simulink model "Lombardini_dual_fuel"  (R2024b)
settings: Solver=FixedStepAuto  StartTime=0.0  StopTime=2000  RelTol=1e-3  EnableMultiTasking=on
PreLoadFcn:
  | try, eval([bdroot '_setup']); catch, eval('model_setup', ''); end
InitFcn:
  | try, eval([bdroot '_setup']); catch, eval('model_setup', ''); end
model workspace (MAT data in the model file):
  PID_rpm = [1000 2000 3000 4000]
undefined symbols (not defined in the file): ECU555, motohawk_build_version, motohawk_get_target_image, motohawk_target_type, motohawk_trunc_name, motohawk_vardec_path
libraries: MotoHawk_lib x118, motohawk_annotations_lib x23, dspstat3 x13, motohawk_examples_lib x1, MotoHawk_Protocols_lib x1
(part 5 of 5)

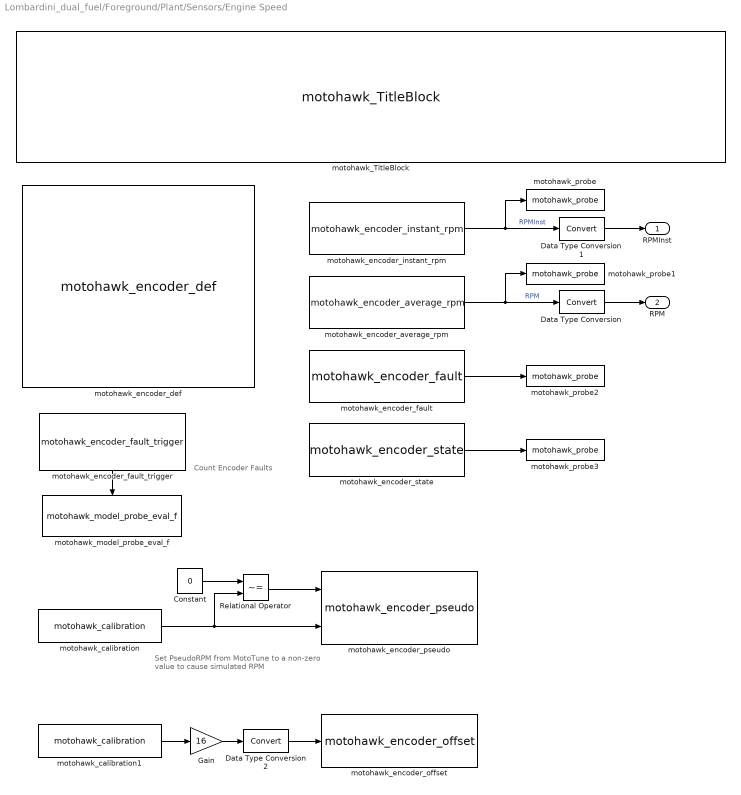
== system Lombardini_dual_fuel/Foreground/Plant/Sensors/Engine Speed ==
  note: Set PseudoRPM from MotoTune
      | to a non-zero value to cause
      | simulated RPM
  note: Count
      | Encoder
      | Faults
  Constant : Constant  Value=0  OutDataTypeStr=Inherit: Inherit via back propagation
  Data Type Conversion : DataTypeConversion
  Data Type Conversion1 : DataTypeConversion
  Data Type Conversion2 : DataTypeConversion
  Gain : Gain  Gain=16  OutDataTypeStr=Inherit: Same as input  ParamDataTypeStr=Inherit: Same as input
  Relational Operator : RelationalOperator  Operator=~=  ZeroCross=off
  motohawk_TitleBlock : motohawk_annotations_lib/motohawk_TitleBlock  BlockType_='Mototron_Title_Block'  ttl=[get_param(bdroot, 'Description') '\rm\newlineEngine Encoder Interface\newlineOutput RPM for use in the controller\newline']  copyright="'THE INFORMATION CONTAINED IN THIS\\newlineDRAWING IS THE SOLE PROPERTY OF\\newlineWOODWARD.  ANY REPRODUCTION IN\\newline PART OR AS A WHOLE WITHOUT THE\\newlineWRITTEN PERMISSION OF WOODWARD\\newline IS PROHIBITED.\\fontsize{16}\\rm\\copyright\\rm\\fontsize{10} 2017'"  address='\fontsize{22}\it\fontname{Arial Black}Woodward \fontname{Arial}\fontsize{10}\newline1081 Woodward Way, Fort Collins, CO, 80524\newlinemcs.woodward.com'  image_file='mh.jpg'  pretty_print=on  edit_text=|  edit_as=6
      | [get_param(bdroot, 'Description') '\rm
      | 
      | 
      | Engine Encoder Interface
      | 
      | 
      | Output RPM for use in the controller
      | 
      | 
      | ']
      settings: SourceProductName=MotoHawk Annotations
  motohawk_calibration : MotoHawk_lib/Calibration & Probing Blocks/motohawk_calibration  name_source=Use Parameter  nam='PseudoRPM'  val=0  storage=Display  ovr_cals=on  data_type=Inherit via back propagation  mem_region_use=off  mem_region_name='SERIAL_EE'  read_level=1  write_level=1  view_as=Number  enum_struct={'Disabled', 'Enabled'}  vector_style=Wide Row  row_header_enum={}  col_header_enum={}  mototune_group=motohawk_vardec_path(gcb)  help=''  units=''  min_val=-inf  max_val=inf  precision=''  gain=1  offset=0  exp=1  show_more=on  use_help_units=off  use_header_enum=off  use_min_max=off  use_precision=off  use_mototune_group=off  data_stores=motohawk_sfun_calibration_data_stores
      settings: SourceProductName=MotoHawk
  motohawk_calibration1 : MotoHawk_lib/Calibration & Probing Blocks/motohawk_calibration  name_source=Use Parameter  nam='EncoderTDCOffset'  val=0  storage=Calibration  ovr_cals=on  data_type=Inherit via back propagation  mem_region_use=off  mem_region_name='SERIAL_EE'  read_level=1  write_level=1  view_as=Number  enum_struct={'Disabled', 'Enabled'}  vector_style=Wide Row  row_header_enum={}  col_header_enum={}  mototune_group='System | Encoder | Encoder Config'  help="'TDC offset of crank sensor, in degrees before TDC1.  Used to align sensor with crank angle.'"  units='degCA'  min_val=0  max_val=720  precision=''  gain=1  offset=0  exp=1  show_more=on  use_help_units=on  use_header_enum=off  use_min_max=on  use_precision=off  use_mototune_group=on  data_stores=motohawk_sfun_calibration_data_stores
      settings: SourceProductName=MotoHawk
  motohawk_encoder_average_rpm : MotoHawk_lib/Encoder Blocks/motohawk_encoder_average_rpm  resolution=1
      settings: SourceProductName=MotoHawk
  motohawk_encoder_def : MotoHawk_lib/Encoder Blocks/motohawk_encoder_def  encoder_type=60 Minus 6 - 4-Stroke - No CAM  interface=VR Crank  sync=Falling Edge  crnkpullup=Weak Pullup  camsync=Rising Edge  campullup=Weak Pullup  angle_offset=0  sec_tdcoffset=-34.3  cam_delay=0  teeth_after_cam=-1  ignore_teeth=0  ignore_delay=0  angles=[0 360 180 540]  cnk_align_with_cam=off  adaptive_vr_cnk=off  adaptive_vr_cam=on  cal_cylinders=on  max_cylinders=8  num_cylinders=4  read_level=1  write_level=1  ovr_cals=on  group='System | Encoder'
      settings: SourceProductName=MotoHawk
  motohawk_encoder_fault : MotoHawk_lib/Encoder Blocks/motohawk_encoder_fault
      settings: SourceProductName=MotoHawk
  motohawk_encoder_fault_trigger : MotoHawk_lib/Encoder Blocks/motohawk_encoder_fault_trigger  Tag=Trigger  trig_name=[]  use_task_name=off  task_priority=ApplicationInterruptTask  task_name='ApplicationInterruptTask'  inherited=off
      settings: SourceProductName=MotoHawk
  motohawk_encoder_instant_rpm : MotoHawk_lib/Encoder Blocks/motohawk_encoder_instant_rpm  resolution=1
      settings: SourceProductName=MotoHawk
  motohawk_encoder_offset : MotoHawk_lib/Encoder Blocks/motohawk_encoder_offset
      settings: SourceProductName=MotoHawk
  motohawk_encoder_pseudo : MotoHawk_lib/Encoder Blocks/motohawk_encoder_pseudo
      settings: SourceProductName=MotoHawk
  motohawk_encoder_state : MotoHawk_lib/Encoder Blocks/motohawk_encoder_state
      settings: SourceProductName=MotoHawk
  motohawk_model_probe_eval_f : MotoHawk_lib/Extra Development Blocks/motohawk_model_probe_eval_f  nam='EncoderFaultCount'  group=motohawk_vardec_path(gcb)
      settings: SourceProductName=MotoHawk
  motohawk_probe : MotoHawk_lib/Calibration & Probing Blocks/motohawk_probe  nam='RPMInst'  show_more=on  name_source=Use Input Wire Name  read_level=1  view_as=Number  enum_struct={'Disabled', 'Enabled'}  vector_style=Wide Row  use_help_units=off  help=''  units=''  use_header_enum=off  row_header_enum={}  col_header_enum={}  use_min_max=off  min_val=-inf  max_val=inf  use_precision=off  precision=''  gain=1  offset=0  exp=1  use_mototune_group=off  mototune_group=motohawk_vardec_path(gcb)
      settings: SourceProductName=MotoHawk
  motohawk_probe1 : MotoHawk_lib/Calibration & Probing Blocks/motohawk_probe  nam='RPM'  show_more=on  name_source=Use Input Wire Name  read_level=1  view_as=Number  enum_struct={'Disabled', 'Enabled'}  vector_style=Wide Row  use_help_units=off  help=''  units=''  use_header_enum=off  row_header_enum={}  col_header_enum={}  use_min_max=off  min_val=-inf  max_val=inf  use_precision=off  precision=''  gain=1  offset=0  exp=1  use_mototune_group=off  mototune_group=motohawk_vardec_path(gcb)
      settings: SourceProductName=MotoHawk
  motohawk_probe2 : MotoHawk_lib/Calibration & Probing Blocks/motohawk_probe  nam='EncoderFault'  show_more=on  name_source=Use Parameter  read_level=1  view_as=Enumeration  enum_struct={'OK', 'Crank Sync Fault', 'Reverse Rotation', 'No Crank Edges', 'No CAM Edges', 'CAM Sync Fault','Encoder Sync Error on Slave','Reverse Rotation on Slave','Slave Encoder Loss'}  vector_style=Wide Row  use_help_units=on  help='Encoder synchronization fault status'  units=''  use_header_enum=off  row_header_enum={}  col_header_enum={}  use_min_max=off  min_val=-inf  max_val=inf  use_precision=off  precision=''  gain=1  offset=0  exp=1  use_mototune_group=off  mototune_group=motohawk_vardec_path(gcb)
      settings: SourceProductName=MotoHawk
  motohawk_probe3 : MotoHawk_lib/Calibration & Probing Blocks/motohawk_probe  nam='EncoderState'  show_more=on  name_source=Use Parameter  read_level=1  view_as=Enumeration  enum_struct={'', 'Zero Speed', 'Position Unknown', 'Crank Sync - CAM Unknown', 'Crank Sync - CAM Sync', 'Crank Sync - Master Only', 'Crank Sync - Slave Only', 'Crank Sync - Master + Slave'}  vector_style=Wide Row  use_help_units=on  help='Encoder synchronization status'  units=''  use_header_enum=off  row_header_enum={}  col_header_enum={}  use_min_max=off  min_val=-inf  max_val=inf  use_precision=off  precision=''  gain=1  offset=0  exp=1  use_mototune_group=off  mototune_group=motohawk_vardec_path(gcb)
      settings: SourceProductName=MotoHawk
  RPMInst : Outport  VectorParamsAs1DForOutWhenUnconnected=off
  RPM : Outport  Port=2  VectorParamsAs1DForOutWhenUnconnected=off
  wires:
  motohawk_encoder_instant_rpm/1 -> motohawk_probe/1, Data Type Conversion1/1  "RPMInst"
  motohawk_encoder_average_rpm/1 -> motohawk_probe1/1, Data Type Conversion/1  "RPM"
  motohawk_calibration/1 -> motohawk_encoder_pseudo/2, Relational Operator/2
  Relational Operator/1 -> motohawk_encoder_pseudo/1
  Constant/1 -> Relational Operator/1
  Data Type Conversion/1 -> RPM/1
  Data Type Conversion1/1 -> RPMInst/1
  motohawk_encoder_fault/1 -> motohawk_probe2/1
  motohawk_calibration1/1 -> Gain/1
  Gain/1 -> Data Type Conversion2/1
  Data Type Conversion2/1 -> motohawk_encoder_offset/1
  motohawk_encoder_state/1 -> motohawk_probe3/1
  motohawk_encoder_fault_trigger/1 -> motohawk_model_probe_eval_f/Trigger

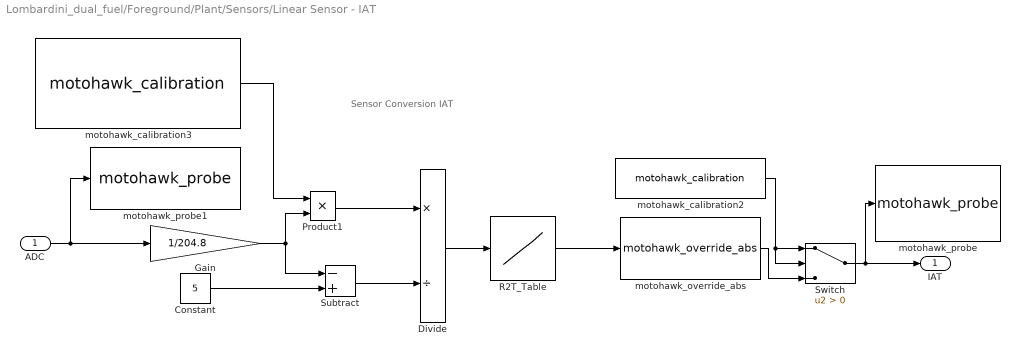
== system Lombardini_dual_fuel/Foreground/Plant/Sensors/Linear Sensor - IAT ==
  note: Sensor Conversion
      | IAT
  ADC : Inport
  Constant : Constant  Value=5
  Divide : Product  Inputs=*/
  Gain : Gain  Gain=1/204.8  OutDataTypeStr=double
  Product1 : Product  InputSameDT=on  OutDataTypeStr=Inherit: Same as first input
  R2T_Table : Lookup_n-D  NumberOfTableDimensions=1  BreakpointsForDimension1=[-5:5]  Table=tanh([-5:5])  InternalRulePriority=Speed  RndMeth=Simplest
  Subtract : Sum  Inputs=-+
  Switch : Switch  Criteria=u2 > Threshold  SaturateOnIntegerOverflow=off  InputSameDT=off
  motohawk_calibration2 : MotoHawk_lib/Calibration & Probing Blocks/motohawk_calibration  name_source=Use Parameter  nam='IAT_Override'  val=25  storage=Calibration  ovr_cals=on  data_type=Inherit from 'Default Value'  mem_region_use=off  mem_region_name='SERIAL_EE'  read_level=1  write_level=1  view_as=Number  enum_struct={'Disabled', 'Enabled'}  vector_style=Wide Row  row_header_enum={}  col_header_enum={}  mototune_group=motohawk_vardec_path(gcb)  help=''  units=''  min_val=-inf  max_val=inf  precision=''  gain=1  offset=0  exp=1  show_more=off  use_help_units=off  use_header_enum=off  use_min_max=off  use_precision=off  use_mototune_group=off  data_stores=motohawk_sfun_calibration_data_stores
      settings: SourceProductName=MotoHawk
  motohawk_calibration3 : MotoHawk_lib/Calibration & Probing Blocks/motohawk_calibration  name_source=Use Parameter  nam='IAT_Calibration_Pullup'  val=1000  storage=Calibration  ovr_cals=on  data_type=Inherit from 'Default Value'  mem_region_use=off  mem_region_name='SERIAL_EE'  read_level=1  write_level=1  view_as=Number  enum_struct={'Disabled', 'Enabled'}  vector_style=Wide Row  row_header_enum={}  col_header_enum={}  mototune_group=motohawk_vardec_path(gcb)  help=''  units=''  min_val=-inf  max_val=inf  precision=''  gain=1  offset=0  exp=1  show_more=off  use_help_units=off  use_header_enum=off  use_min_max=off  use_precision=off  use_mototune_group=off  data_stores=motohawk_sfun_calibration_data_stores
      settings: SourceProductName=MotoHawk
  motohawk_override_abs : MotoHawk_lib/Calibration & Probing Blocks/motohawk_override_abs  parent_name='IAT'  parent_val=0  show_more=off  name_source=Use Parameter  parent_read_level=1  parent_override_level=1  view_as=Number  enum_struct={'Disabled', 'Enabled'}  use_help_units=off  parent_help=''  parent_units=''  use_min_max=off  parent_min=-inf  parent_max=inf  use_precision=off  parent_precision=''  parent_gain=1  parent_offset=0  parent_exp=1  use_mototune_group=off  parent_group=motohawk_vardec_path(gcb)
      settings: SourceProductName=MotoHawk
  motohawk_probe : MotoHawk_lib/Calibration & Probing Blocks/motohawk_probe  nam='IAT_postc'  show_more=off  name_source=Use Parameter  read_level=1  view_as=Number  enum_struct={'Disabled', 'Enabled'}  vector_style=Wide Row  use_help_units=off  help=''  units=''  use_header_enum=off  row_header_enum={}  col_header_enum={}  use_min_max=off  min_val=-inf  max_val=inf  use_precision=off  precision=''  gain=1  offset=0  exp=1  use_mototune_group=off  mototune_group=motohawk_vardec_path(gcb)
      settings: SourceProductName=MotoHawk
  motohawk_probe1 : MotoHawk_lib/Calibration & Probing Blocks/motohawk_probe  nam='IAT'  show_more=off  name_source=Use Parameter  read_level=1  view_as=Number  enum_struct={'Disabled', 'Enabled'}  vector_style=Wide Row  use_help_units=off  help=''  units=''  use_header_enum=off  row_header_enum={}  col_header_enum={}  use_min_max=off  min_val=-inf  max_val=inf  use_precision=off  precision=''  gain=1  offset=0  exp=1  use_mototune_group=off  mototune_group=motohawk_vardec_path(gcb)
      settings: SourceProductName=MotoHawk
  IAT : Outport  VectorParamsAs1DForOutWhenUnconnected=off
  wires:
  Gain/1 -> Subtract/1, Product1/2
  ADC/1 -> Gain/1, motohawk_probe1/1
  Divide/1 -> R2T_Table/1
  Switch/1 -> motohawk_probe/1, IAT/1
  motohawk_calibration2/1 -> Switch/2, Switch/1
  motohawk_override_abs/1 -> Switch/3
  motohawk_calibration3/1 -> Product1/1
  Constant/1 -> Subtract/2
  Subtract/1 -> Divide/2
  Product1/1 -> Divide/1
  R2T_Table/1 -> motohawk_override_abs/1

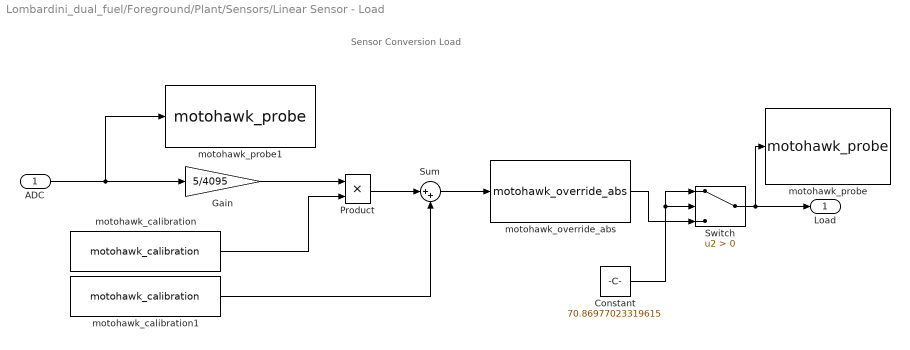
== system Lombardini_dual_fuel/Foreground/Plant/Sensors/Linear Sensor - Load ==
  note: Sensor Conversion
      | Load
  ADC : Inport
  Constant : Constant  Value=70.86977023319615  OutDataTypeStr=single
  Gain : Gain  Gain=5/4095  ParamDataTypeStr=double
  Product : Product  InputSameDT=on  OutDataTypeStr=Inherit: Same as first input
  Sum : Sum  Inputs=|++  InputSameDT=on
  Switch : Switch  Criteria=u2 > Threshold  SaturateOnIntegerOverflow=off  InputSameDT=off
  motohawk_calibration : MotoHawk_lib/Calibration & Probing Blocks/motohawk_calibration  name_source=Use Parameter  nam='Load_Gain'  val=1  storage=Calibration  ovr_cals=on  data_type=Inherit from 'Default Value'  mem_region_use=off  mem_region_name='SERIAL_EE'  read_level=1  write_level=1  view_as=Number  enum_struct={'Disabled', 'Enabled'}  vector_style=Wide Row  row_header_enum={}  col_header_enum={}  mototune_group=motohawk_vardec_path(gcb)  help=''  units=''  min_val=-inf  max_val=inf  precision=''  gain=1  offset=0  exp=1  show_more=off  use_help_units=off  use_header_enum=off  use_min_max=off  use_precision=off  use_mototune_group=off  data_stores=motohawk_sfun_calibration_data_stores
      settings: SourceProductName=MotoHawk
  motohawk_calibration1 : MotoHawk_lib/Calibration & Probing Blocks/motohawk_calibration  name_source=Use Parameter  nam='Load_Offset'  val=0  storage=Calibration  ovr_cals=on  data_type=Inherit from 'Default Value'  mem_region_use=off  mem_region_name='SERIAL_EE'  read_level=1  write_level=1  view_as=Number  enum_struct={'Disabled', 'Enabled'}  vector_style=Wide Row  row_header_enum={}  col_header_enum={}  mototune_group=motohawk_vardec_path(gcb)  help=''  units=''  min_val=-inf  max_val=inf  precision=''  gain=1  offset=0  exp=1  show_more=off  use_help_units=off  use_header_enum=off  use_min_max=off  use_precision=off  use_mototune_group=off  data_stores=motohawk_sfun_calibration_data_stores
      settings: SourceProductName=MotoHawk
  motohawk_override_abs : MotoHawk_lib/Calibration & Probing Blocks/motohawk_override_abs  parent_name='Load'  parent_val=0  show_more=off  name_source=Use Parameter  parent_read_level=1  parent_override_level=1  view_as=Number  enum_struct={'Disabled', 'Enabled'}  use_help_units=off  parent_help=''  parent_units=''  use_min_max=off  parent_min=-inf  parent_max=inf  use_precision=off  parent_precision=''  parent_gain=1  parent_offset=0  parent_exp=1  use_mototune_group=off  parent_group=motohawk_vardec_path(gcb)
      settings: SourceProductName=MotoHawk
  motohawk_probe : MotoHawk_lib/Calibration & Probing Blocks/motohawk_probe  nam='Load_postc'  show_more=off  name_source=Use Parameter  read_level=1  view_as=Number  enum_struct={'Disabled', 'Enabled'}  vector_style=Wide Row  use_help_units=off  help=''  units=''  use_header_enum=off  row_header_enum={}  col_header_enum={}  use_min_max=off  min_val=-inf  max_val=inf  use_precision=off  precision=''  gain=1  offset=0  exp=1  use_mototune_group=off  mototune_group=motohawk_vardec_path(gcb)
      settings: SourceProductName=MotoHawk
  motohawk_probe1 : MotoHawk_lib/Calibration & Probing Blocks/motohawk_probe  nam='Load'  show_more=off  name_source=Use Parameter  read_level=1  view_as=Number  enum_struct={'Disabled', 'Enabled'}  vector_style=Wide Row  use_help_units=off  help=''  units=''  use_header_enum=off  row_header_enum={}  col_header_enum={}  use_min_max=off  min_val=-inf  max_val=inf  use_precision=off  precision=''  gain=1  offset=0  exp=1  use_mototune_group=off  mototune_group=motohawk_vardec_path(gcb)
      settings: SourceProductName=MotoHawk
  Load : Outport  VectorParamsAs1DForOutWhenUnconnected=off
  wires:
  motohawk_calibration/1 -> Product/2
  Product/1 -> Sum/1
  motohawk_calibration1/1 -> Sum/2
  Gain/1 -> Product/1
  ADC/1 -> Gain/1, motohawk_probe1/1
  Sum/1 -> motohawk_override_abs/1
  Switch/1 -> motohawk_probe/1, Load/1
  Constant/1 -> Switch/1, Switch/2
  motohawk_override_abs/1 -> Switch/3

== system Lombardini_dual_fuel/Foreground/Plant/Sensors/Linear Sensor - MAP ==
  note: Sensor Conversion
      | MAP
  ADC : Inport
  Data Type Conversion : DataTypeConversion  OutDataTypeStr=double  SaturateOnIntegerOverflow=off  RndMeth=Floor
  Gain : Gain  Gain=single(5/4095)
  Product : Product  InputSameDT=on  OutDataTypeStr=Inherit: Same as first input
  Sum : Sum  Inputs=|++  InputSameDT=on
  motohawk_calibration : MotoHawk_lib/Calibration & Probing Blocks/motohawk_calibration  name_source=Use Parameter  nam='MAP_Gain'  val=1  storage=Calibration  ovr_cals=on  data_type=Inherit from 'Default Value'  mem_region_use=off  mem_region_name='SERIAL_EE'  read_level=1  write_level=1  view_as=Number  enum_struct={'Disabled', 'Enabled'}  vector_style=Wide Row  row_header_enum={}  col_header_enum={}  mototune_group=motohawk_vardec_path(gcb)  help=''  units=''  min_val=-inf  max_val=inf  precision=''  gain=1  offset=0  exp=1  show_more=off  use_help_units=off  use_header_enum=off  use_min_max=off  use_precision=off  use_mototune_group=off  data_stores=motohawk_sfun_calibration_data_stores
      settings: SourceProductName=MotoHawk
  motohawk_calibration1 : MotoHawk_lib/Calibration & Probing Blocks/motohawk_calibration  name_source=Use Parameter  nam='MAP_Offset'  val=0  storage=Calibration  ovr_cals=on  data_type=Inherit from 'Default Value'  mem_region_use=off  mem_region_name='SERIAL_EE'  read_level=1  write_level=1  view_as=Number  enum_struct={'Disabled', 'Enabled'}  vector_style=Wide Row  row_header_enum={}  col_header_enum={}  mototune_group=motohawk_vardec_path(gcb)  help=''  units=''  min_val=-inf  max_val=inf  precision=''  gain=1  offset=0  exp=1  show_more=off  use_help_units=off  use_header_enum=off  use_min_max=off  use_precision=off  use_mototune_group=off  data_stores=motohawk_sfun_calibration_data_stores
      settings: SourceProductName=MotoHawk
  motohawk_override_abs : MotoHawk_lib/Calibration & Probing Blocks/motohawk_override_abs  parent_name='MAP'  parent_val=1  show_more=off  name_source=Use Parameter  parent_read_level=1  parent_override_level=1  view_as=Number  enum_struct={'Disabled', 'Enabled'}  use_help_units=off  parent_help=''  parent_units=''  use_min_max=off  parent_min=-inf  parent_max=inf  use_precision=off  parent_precision=''  parent_gain=1  parent_offset=0  parent_exp=1  use_mototune_group=off  parent_group=motohawk_vardec_path(gcb)
      settings: SourceProductName=MotoHawk
  motohawk_probe : MotoHawk_lib/Calibration & Probing Blocks/motohawk_probe  nam='MAP'  show_more=off  name_source=Use Parameter  read_level=1  view_as=Number  enum_struct={'Disabled', 'Enabled'}  vector_style=Wide Row  use_help_units=off  help=''  units=''  use_header_enum=off  row_header_enum={}  col_header_enum={}  use_min_max=off  min_val=-inf  max_val=inf  use_precision=off  precision=''  gain=1  offset=0  exp=1  use_mototune_group=off  mototune_group=motohawk_vardec_path(gcb)
      settings: SourceProductName=MotoHawk
  motohawk_probe1 : MotoHawk_lib/Calibration & Probing Blocks/motohawk_probe  nam='MAP_ADC'  show_more=off  name_source=Use Parameter  read_level=1  view_as=Number  enum_struct={'Disabled', 'Enabled'}  vector_style=Wide Row  use_help_units=off  help=''  units=''  use_header_enum=off  row_header_enum={}  col_header_enum={}  use_min_max=off  min_val=-inf  max_val=inf  use_precision=off  precision=''  gain=1  offset=0  exp=1  use_mototune_group=off  mototune_group=motohawk_vardec_path(gcb)
      settings: SourceProductName=MotoHawk
  MAP : Outport  VectorParamsAs1DForOutWhenUnconnected=off
  wires:
  motohawk_calibration/1 -> Product/2
  Product/1 -> Sum/1
  motohawk_calibration1/1 -> Sum/2
  Gain/1 -> Data Type Conversion/1
  ADC/1 -> Gain/1, motohawk_probe1/1
  Sum/1 -> motohawk_override_abs/1
  motohawk_override_abs/1 -> MAP/1, motohawk_probe/1
  Data Type Conversion/1 -> Product/1

== system Lombardini_dual_fuel/Foreground/Plant/Sensors/Linear Sensor - P_Baro ==
  note: Sensor Conversion
      | P_Baro
  ADC : Inport
  Gain : Gain  Gain=5/4095  OutDataTypeStr=double
  Product : Product  InputSameDT=on  OutDataTypeStr=Inherit: Same as first input
  Sum : Sum  Inputs=|++  InputSameDT=on
  motohawk_calibration : MotoHawk_lib/Calibration & Probing Blocks/motohawk_calibration  name_source=Use Parameter  nam='P_Baro_Gain'  val=1  storage=Calibration  ovr_cals=on  data_type=Inherit from 'Default Value'  mem_region_use=off  mem_region_name='SERIAL_EE'  read_level=1  write_level=1  view_as=Number  enum_struct={'Disabled', 'Enabled'}  vector_style=Wide Row  row_header_enum={}  col_header_enum={}  mototune_group=motohawk_vardec_path(gcb)  help=''  units=''  min_val=-inf  max_val=inf  precision=''  gain=1  offset=0  exp=1  show_more=off  use_help_units=off  use_header_enum=off  use_min_max=off  use_precision=off  use_mototune_group=off  data_stores=motohawk_sfun_calibration_data_stores
      settings: SourceProductName=MotoHawk
  motohawk_calibration1 : MotoHawk_lib/Calibration & Probing Blocks/motohawk_calibration  name_source=Use Parameter  nam='P_Baro_Offset'  val=0  storage=Calibration  ovr_cals=on  data_type=Inherit from 'Default Value'  mem_region_use=off  mem_region_name='SERIAL_EE'  read_level=1  write_level=1  view_as=Number  enum_struct={'Disabled', 'Enabled'}  vector_style=Wide Row  row_header_enum={}  col_header_enum={}  mototune_group=motohawk_vardec_path(gcb)  help=''  units=''  min_val=-inf  max_val=inf  precision=''  gain=1  offset=0  exp=1  show_more=off  use_help_units=off  use_header_enum=off  use_min_max=off  use_precision=off  use_mototune_group=off  data_stores=motohawk_sfun_calibration_data_stores
      settings: SourceProductName=MotoHawk
  motohawk_override_abs : MotoHawk_lib/Calibration & Probing Blocks/motohawk_override_abs  parent_name='P_Baro'  parent_val=1  show_more=off  name_source=Use Parameter  parent_read_level=1  parent_override_level=1  view_as=Number  enum_struct={'Disabled', 'Enabled'}  use_help_units=off  parent_help=''  parent_units=''  use_min_max=off  parent_min=-inf  parent_max=inf  use_precision=off  parent_precision=''  parent_gain=1  parent_offset=0  parent_exp=1  use_mototune_group=off  parent_group=motohawk_vardec_path(gcb)
      settings: SourceProductName=MotoHawk
  motohawk_probe : MotoHawk_lib/Calibration & Probing Blocks/motohawk_probe  nam='P_Baro_postc'  show_more=off  name_source=Use Parameter  read_level=1  view_as=Number  enum_struct={'Disabled', 'Enabled'}  vector_style=Wide Row  use_help_units=off  help=''  units=''  use_header_enum=off  row_header_enum={}  col_header_enum={}  use_min_max=off  min_val=-inf  max_val=inf  use_precision=off  precision=''  gain=1  offset=0  exp=1  use_mototune_group=off  mototune_group=motohawk_vardec_path(gcb)
      settings: SourceProductName=MotoHawk
  motohawk_probe1 : MotoHawk_lib/Calibration & Probing Blocks/motohawk_probe  nam='P_Baro'  show_more=off  name_source=Use Parameter  read_level=1  view_as=Number  enum_struct={'Disabled', 'Enabled'}  vector_style=Wide Row  use_help_units=off  help=''  units=''  use_header_enum=off  row_header_enum={}  col_header_enum={}  use_min_max=off  min_val=-inf  max_val=inf  use_precision=off  precision=''  gain=1  offset=0  exp=1  use_mototune_group=off  mototune_group=motohawk_vardec_path(gcb)
      settings: SourceProductName=MotoHawk
  P_Baro : Outport  VectorParamsAs1DForOutWhenUnconnected=off
  wires:
  motohawk_calibration/1 -> Product/2
  Product/1 -> Sum/1
  motohawk_calibration1/1 -> Sum/2
  Gain/1 -> Product/1
  ADC/1 -> Gain/1, motohawk_probe1/1
  Sum/1 -> motohawk_override_abs/1
  motohawk_override_abs/1 -> motohawk_probe/1, P_Baro/1

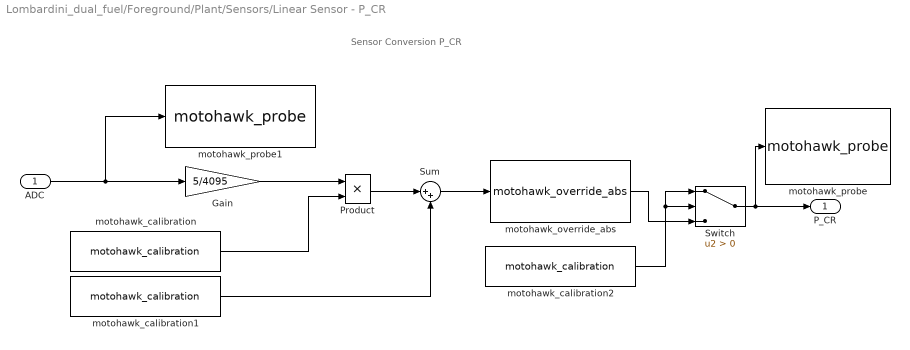
== system Lombardini_dual_fuel/Foreground/Plant/Sensors/Linear Sensor - P_CR ==
  note: Sensor Conversion
      | P_CR
  ADC : Inport
  Gain : Gain  Gain=5/4095  OutDataTypeStr=double
  Product : Product  InputSameDT=on  OutDataTypeStr=Inherit: Same as first input
  Sum : Sum  Inputs=|++  InputSameDT=on
  Switch : Switch  Criteria=u2 > Threshold  SaturateOnIntegerOverflow=off  InputSameDT=off
  motohawk_calibration : MotoHawk_lib/Calibration & Probing Blocks/motohawk_calibration  name_source=Use Parameter  nam='P_CR_Gain'  val=1  storage=Calibration  ovr_cals=on  data_type=Inherit from 'Default Value'  mem_region_use=off  mem_region_name='SERIAL_EE'  read_level=1  write_level=1  view_as=Number  enum_struct={'Disabled', 'Enabled'}  vector_style=Wide Row  row_header_enum={}  col_header_enum={}  mototune_group=motohawk_vardec_path(gcb)  help=''  units=''  min_val=-inf  max_val=inf  precision=''  gain=1  offset=0  exp=1  show_more=off  use_help_units=off  use_header_enum=off  use_min_max=off  use_precision=off  use_mototune_group=off  data_stores=motohawk_sfun_calibration_data_stores
      settings: SourceProductName=MotoHawk
  motohawk_calibration1 : MotoHawk_lib/Calibration & Probing Blocks/motohawk_calibration  name_source=Use Parameter  nam='P_CR_Offset'  val=0  storage=Calibration  ovr_cals=on  data_type=Inherit from 'Default Value'  mem_region_use=off  mem_region_name='SERIAL_EE'  read_level=1  write_level=1  view_as=Number  enum_struct={'Disabled', 'Enabled'}  vector_style=Wide Row  row_header_enum={}  col_header_enum={}  mototune_group=motohawk_vardec_path(gcb)  help=''  units=''  min_val=-inf  max_val=inf  precision=''  gain=1  offset=0  exp=1  show_more=off  use_help_units=off  use_header_enum=off  use_min_max=off  use_precision=off  use_mototune_group=off  data_stores=motohawk_sfun_calibration_data_stores
      settings: SourceProductName=MotoHawk
  motohawk_calibration2 : MotoHawk_lib/Calibration & Probing Blocks/motohawk_calibration  name_source=Use Parameter  nam='P_CR_Override'  val=100  storage=Calibration  ovr_cals=on  data_type=Inherit from 'Default Value'  mem_region_use=off  mem_region_name='SERIAL_EE'  read_level=1  write_level=1  view_as=Number  enum_struct={'Disabled', 'Enabled'}  vector_style=Wide Row  row_header_enum={}  col_header_enum={}  mototune_group=motohawk_vardec_path(gcb)  help=''  units=''  min_val=-inf  max_val=inf  precision=''  gain=1  offset=0  exp=1  show_more=off  use_help_units=off  use_header_enum=off  use_min_max=off  use_precision=off  use_mototune_group=off  data_stores=motohawk_sfun_calibration_data_stores
      settings: SourceProductName=MotoHawk
  motohawk_override_abs : MotoHawk_lib/Calibration & Probing Blocks/motohawk_override_abs  parent_name='P_CR'  parent_val=0  show_more=off  name_source=Use Parameter  parent_read_level=1  parent_override_level=1  view_as=Number  enum_struct={'Disabled', 'Enabled'}  use_help_units=off  parent_help=''  parent_units=''  use_min_max=off  parent_min=-inf  parent_max=inf  use_precision=off  parent_precision=''  parent_gain=1  parent_offset=0  parent_exp=1  use_mototune_group=off  parent_group=motohawk_vardec_path(gcb)
      settings: SourceProductName=MotoHawk
  motohawk_probe : MotoHawk_lib/Calibration & Probing Blocks/motohawk_probe  nam='P_CR_post'  show_more=off  name_source=Use Parameter  read_level=1  view_as=Number  enum_struct={'Disabled', 'Enabled'}  vector_style=Wide Row  use_help_units=off  help=''  units=''  use_header_enum=off  row_header_enum={}  col_header_enum={}  use_min_max=off  min_val=-inf  max_val=inf  use_precision=off  precision=''  gain=1  offset=0  exp=1  use_mototune_group=off  mototune_group=motohawk_vardec_path(gcb)
      settings: SourceProductName=MotoHawk
  motohawk_probe1 : MotoHawk_lib/Calibration & Probing Blocks/motohawk_probe  nam='P_CR'  show_more=off  name_source=Use Parameter  read_level=1  view_as=Number  enum_struct={'Disabled', 'Enabled'}  vector_style=Wide Row  use_help_units=off  help=''  units=''  use_header_enum=off  row_header_enum={}  col_header_enum={}  use_min_max=off  min_val=-inf  max_val=inf  use_precision=off  precision=''  gain=1  offset=0  exp=1  use_mototune_group=off  mototune_group=motohawk_vardec_path(gcb)
      settings: SourceProductName=MotoHawk
  P_CR : Outport  VectorParamsAs1DForOutWhenUnconnected=off
  wires:
  motohawk_calibration/1 -> Product/2
  Product/1 -> Sum/1
  motohawk_calibration1/1 -> Sum/2
  Gain/1 -> Product/1
  ADC/1 -> Gain/1, motohawk_probe1/1
  Sum/1 -> motohawk_override_abs/1
  Switch/1 -> motohawk_probe/1, P_CR/1
  motohawk_calibration2/1 -> Switch/1, Switch/2
  motohawk_override_abs/1 -> Switch/3

== system Lombardini_dual_fuel/Foreground/Plant/Sensors/Linear Sensor - P_Fuel ==
  note: Sensor Conversion
      | P_Fuel
  ADC : Inport
  Gain : Gain  Gain=5/4095  OutDataTypeStr=double
  Product : Product  InputSameDT=on  OutDataTypeStr=Inherit: Same as first input
  Sum : Sum  Inputs=|++  InputSameDT=on
  motohawk_calibration : MotoHawk_lib/Calibration & Probing Blocks/motohawk_calibration  name_source=Use Parameter  nam='P_Fuel_Gain'  val=1  storage=Calibration  ovr_cals=on  data_type=Inherit from 'Default Value'  mem_region_use=off  mem_region_name='SERIAL_EE'  read_level=1  write_level=1  view_as=Number  enum_struct={'Disabled', 'Enabled'}  vector_style=Wide Row  row_header_enum={}  col_header_enum={}  mototune_group=motohawk_vardec_path(gcb)  help=''  units=''  min_val=-inf  max_val=inf  precision=''  gain=1  offset=0  exp=1  show_more=off  use_help_units=off  use_header_enum=off  use_min_max=off  use_precision=off  use_mototune_group=off  data_stores=motohawk_sfun_calibration_data_stores
      settings: SourceProductName=MotoHawk
  motohawk_calibration1 : MotoHawk_lib/Calibration & Probing Blocks/motohawk_calibration  name_source=Use Parameter  nam='P_Fuel_Offset'  val=0  storage=Calibration  ovr_cals=on  data_type=Inherit from 'Default Value'  mem_region_use=off  mem_region_name='SERIAL_EE'  read_level=1  write_level=1  view_as=Number  enum_struct={'Disabled', 'Enabled'}  vector_style=Wide Row  row_header_enum={}  col_header_enum={}  mototune_group=motohawk_vardec_path(gcb)  help=''  units=''  min_val=-inf  max_val=inf  precision=''  gain=1  offset=0  exp=1  show_more=off  use_help_units=off  use_header_enum=off  use_min_max=off  use_precision=off  use_mototune_group=off  data_stores=motohawk_sfun_calibration_data_stores
      settings: SourceProductName=MotoHawk
  motohawk_override_abs : MotoHawk_lib/Calibration & Probing Blocks/motohawk_override_abs  parent_name='P_Fuel'  parent_val=5  show_more=off  name_source=Use Parameter  parent_read_level=1  parent_override_level=1  view_as=Number  enum_struct={'Disabled', 'Enabled'}  use_help_units=off  parent_help=''  parent_units=''  use_min_max=off  parent_min=-inf  parent_max=inf  use_precision=off  parent_precision=''  parent_gain=1  parent_offset=0  parent_exp=1  use_mototune_group=off  parent_group=motohawk_vardec_path(gcb)
      settings: SourceProductName=MotoHawk
  motohawk_probe : MotoHawk_lib/Calibration & Probing Blocks/motohawk_probe  nam='P_Fuel_postc'  show_more=off  name_source=Use Parameter  read_level=1  view_as=Number  enum_struct={'Disabled', 'Enabled'}  vector_style=Wide Row  use_help_units=off  help=''  units=''  use_header_enum=off  row_header_enum={}  col_header_enum={}  use_min_max=off  min_val=-inf  max_val=inf  use_precision=off  precision=''  gain=1  offset=0  exp=1  use_mototune_group=off  mototune_group=motohawk_vardec_path(gcb)
      settings: SourceProductName=MotoHawk
  motohawk_probe1 : MotoHawk_lib/Calibration & Probing Blocks/motohawk_probe  nam='P_Fuel'  show_more=off  name_source=Use Parameter  read_level=1  view_as=Number  enum_struct={'Disabled', 'Enabled'}  vector_style=Wide Row  use_help_units=off  help=''  units=''  use_header_enum=off  row_header_enum={}  col_header_enum={}  use_min_max=off  min_val=-inf  max_val=inf  use_precision=off  precision=''  gain=1  offset=0  exp=1  use_mototune_group=off  mototune_group=motohawk_vardec_path(gcb)
      settings: SourceProductName=MotoHawk
  P_Fuel : Outport  VectorParamsAs1DForOutWhenUnconnected=off
  wires:
  motohawk_calibration/1 -> Product/2
  Product/1 -> Sum/1
  motohawk_calibration1/1 -> Sum/2
  Gain/1 -> Product/1
  ADC/1 -> Gain/1, motohawk_probe1/1
  Sum/1 -> motohawk_override_abs/1
  motohawk_override_abs/1 -> motohawk_probe/1, P_Fuel/1

== system Lombardini_dual_fuel/Foreground/Plant/Sensors/Linear Sensor - P_H2 ==
  note: Sensor Conversion
      | P_H2
  ADC : Inport
  Gain : Gain  Gain=5/4095  OutDataTypeStr=double
  Product : Product  InputSameDT=on
  Sum : Sum  Inputs=|++  InputSameDT=on
  motohawk_calibration : MotoHawk_lib/Calibration & Probing Blocks/motohawk_calibration  name_source=Use Parameter  nam='P_H2_Gain'  val=1  storage=Calibration  ovr_cals=on  data_type=double  mem_region_use=off  mem_region_name='SERIAL_EE'  read_level=1  write_level=1  view_as=Number  enum_struct={'Disabled', 'Enabled'}  vector_style=Wide Row  row_header_enum={}  col_header_enum={}  mototune_group=motohawk_vardec_path(gcb)  help=''  units=''  min_val=-inf  max_val=inf  precision=''  gain=1  offset=0  exp=1  show_more=off  use_help_units=off  use_header_enum=off  use_min_max=off  use_precision=off  use_mototune_group=off  data_stores=motohawk_sfun_calibration_data_stores
      settings: SourceProductName=MotoHawk
  motohawk_calibration1 : MotoHawk_lib/Calibration & Probing Blocks/motohawk_calibration  name_source=Use Parameter  nam='P_H2_Offset'  val=0  storage=Calibration  ovr_cals=on  data_type=double  mem_region_use=off  mem_region_name='SERIAL_EE'  read_level=1  write_level=1  view_as=Number  enum_struct={'Disabled', 'Enabled'}  vector_style=Wide Row  row_header_enum={}  col_header_enum={}  mototune_group=motohawk_vardec_path(gcb)  help=''  units=''  min_val=-inf  max_val=inf  precision=''  gain=1  offset=0  exp=1  show_more=off  use_help_units=off  use_header_enum=off  use_min_max=off  use_precision=off  use_mototune_group=off  data_stores=motohawk_sfun_calibration_data_stores
      settings: SourceProductName=MotoHawk
  motohawk_override_abs : MotoHawk_lib/Calibration & Probing Blocks/motohawk_override_abs  parent_name='P_H2'  parent_val=0  show_more=off  name_source=Use Parameter  parent_read_level=1  parent_override_level=1  view_as=Number  enum_struct={'Disabled', 'Enabled'}  use_help_units=off  parent_help=''  parent_units=''  use_min_max=off  parent_min=-inf  parent_max=inf  use_precision=off  parent_precision=''  parent_gain=1  parent_offset=0  parent_exp=1  use_mototune_group=off  parent_group=motohawk_vardec_path(gcb)
      settings: SourceProductName=MotoHawk
  motohawk_probe : MotoHawk_lib/Calibration & Probing Blocks/motohawk_probe  nam='P_H2'  show_more=off  name_source=Use Parameter  read_level=1  view_as=Number  enum_struct={'Disabled', 'Enabled'}  vector_style=Wide Row  use_help_units=off  help=''  units=''  use_header_enum=off  row_header_enum={}  col_header_enum={}  use_min_max=off  min_val=-inf  max_val=inf  use_precision=off  precision=''  gain=1  offset=0  exp=1  use_mototune_group=off  mototune_group=motohawk_vardec_path(gcb)
      settings: SourceProductName=MotoHawk
  motohawk_probe1 : MotoHawk_lib/Calibration & Probing Blocks/motohawk_probe  nam='P_H2_ADC'  show_more=off  name_source=Use Parameter  read_level=1  view_as=Number  enum_struct={'Disabled', 'Enabled'}  vector_style=Wide Row  use_help_units=off  help=''  units=''  use_header_enum=off  row_header_enum={}  col_header_enum={}  use_min_max=off  min_val=-inf  max_val=inf  use_precision=off  precision=''  gain=1  offset=0  exp=1  use_mototune_group=off  mototune_group=motohawk_vardec_path(gcb)
      settings: SourceProductName=MotoHawk
  P_H2 : Outport  VectorParamsAs1DForOutWhenUnconnected=off
  wires:
  motohawk_calibration/1 -> Product/2
  Product/1 -> Sum/1
  motohawk_calibration1/1 -> Sum/2
  Gain/1 -> Product/1
  ADC/1 -> Gain/1, motohawk_probe1/1
  Sum/1 -> motohawk_override_abs/1
  motohawk_override_abs/1 -> P_H2/1, motohawk_probe/1

== system Lombardini_dual_fuel/Foreground/Plant/Sensors/Linear Sensor - T_H2 ==
  note: Sensor Conversion
      | T_H2
  ADC : Inport
  Gain : Gain  Gain=5/4095  OutDataTypeStr=double
  Product : Product  InputSameDT=on  OutDataTypeStr=Inherit: Same as first input
  Sum : Sum  Inputs=|++  InputSameDT=on
  motohawk_calibration : MotoHawk_lib/Calibration & Probing Blocks/motohawk_calibration  name_source=Use Parameter  nam='T_H2_Gain'  val=1  storage=Calibration  ovr_cals=on  data_type=Inherit from 'Default Value'  mem_region_use=off  mem_region_name='SERIAL_EE'  read_level=1  write_level=1  view_as=Number  enum_struct={'Disabled', 'Enabled'}  vector_style=Wide Row  row_header_enum={}  col_header_enum={}  mototune_group=motohawk_vardec_path(gcb)  help=''  units=''  min_val=-inf  max_val=inf  precision=''  gain=1  offset=0  exp=1  show_more=off  use_help_units=off  use_header_enum=off  use_min_max=off  use_precision=off  use_mototune_group=off  data_stores=motohawk_sfun_calibration_data_stores
      settings: SourceProductName=MotoHawk
  motohawk_calibration1 : MotoHawk_lib/Calibration & Probing Blocks/motohawk_calibration  name_source=Use Parameter  nam='T_H2_Offset'  val=0  storage=Calibration  ovr_cals=on  data_type=Inherit from 'Default Value'  mem_region_use=off  mem_region_name='SERIAL_EE'  read_level=1  write_level=1  view_as=Number  enum_struct={'Disabled', 'Enabled'}  vector_style=Wide Row  row_header_enum={}  col_header_enum={}  mototune_group=motohawk_vardec_path(gcb)  help=''  units=''  min_val=-inf  max_val=inf  precision=''  gain=1  offset=0  exp=1  show_more=off  use_help_units=off  use_header_enum=off  use_min_max=off  use_precision=off  use_mototune_group=off  data_stores=motohawk_sfun_calibration_data_stores
      settings: SourceProductName=MotoHawk
  motohawk_override_abs : MotoHawk_lib/Calibration & Probing Blocks/motohawk_override_abs  parent_name='T_H2'  parent_val=0  show_more=off  name_source=Use Parameter  parent_read_level=1  parent_override_level=1  view_as=Number  enum_struct={'Disabled', 'Enabled'}  use_help_units=off  parent_help=''  parent_units=''  use_min_max=off  parent_min=-inf  parent_max=inf  use_precision=off  parent_precision=''  parent_gain=1  parent_offset=0  parent_exp=1  use_mototune_group=off  parent_group=motohawk_vardec_path(gcb)
      settings: SourceProductName=MotoHawk
  motohawk_probe : MotoHawk_lib/Calibration & Probing Blocks/motohawk_probe  nam='T_H2_postc'  show_more=off  name_source=Use Parameter  read_level=1  view_as=Number  enum_struct={'Disabled', 'Enabled'}  vector_style=Wide Row  use_help_units=off  help=''  units=''  use_header_enum=off  row_header_enum={}  col_header_enum={}  use_min_max=off  min_val=-inf  max_val=inf  use_precision=off  precision=''  gain=1  offset=0  exp=1  use_mototune_group=off  mototune_group=motohawk_vardec_path(gcb)
      settings: SourceProductName=MotoHawk
  motohawk_probe1 : MotoHawk_lib/Calibration & Probing Blocks/motohawk_probe  nam='T_H2'  show_more=off  name_source=Use Parameter  read_level=1  view_as=Number  enum_struct={'Disabled', 'Enabled'}  vector_style=Wide Row  use_help_units=off  help=''  units=''  use_header_enum=off  row_header_enum={}  col_header_enum={}  use_min_max=off  min_val=-inf  max_val=inf  use_precision=off  precision=''  gain=1  offset=0  exp=1  use_mototune_group=off  mototune_group=motohawk_vardec_path(gcb)
      settings: SourceProductName=MotoHawk
  T_H2 : Outport  VectorParamsAs1DForOutWhenUnconnected=off
  wires:
  motohawk_calibration/1 -> Product/2
  Product/1 -> Sum/1
  motohawk_calibration1/1 -> Sum/2
  Gain/1 -> Product/1
  ADC/1 -> Gain/1, motohawk_probe1/1
  Sum/1 -> motohawk_override_abs/1
  motohawk_override_abs/1 -> motohawk_probe/1, T_H2/1

== system Lombardini_dual_fuel/Foreground/Plant/Sensors/Linear Sensor - U_Bat ==
  note: Sensor Conversion
      | U_bat
  ADC : Inport
  Gain : Gain  Gain=18/4095  OutDataTypeStr=double
  Product : Product  InputSameDT=on  OutDataTypeStr=Inherit: Same as first input
  Sum : Sum  Inputs=|++  InputSameDT=on
  motohawk_calibration : MotoHawk_lib/Calibration & Probing Blocks/motohawk_calibration  name_source=Use Parameter  nam='U_Bat_Gain'  val=1  storage=Calibration  ovr_cals=on  data_type=Inherit from 'Default Value'  mem_region_use=off  mem_region_name='SERIAL_EE'  read_level=1  write_level=1  view_as=Number  enum_struct={'Disabled', 'Enabled'}  vector_style=Wide Row  row_header_enum={}  col_header_enum={}  mototune_group=motohawk_vardec_path(gcb)  help=''  units=''  min_val=-inf  max_val=inf  precision=''  gain=1  offset=0  exp=1  show_more=off  use_help_units=off  use_header_enum=off  use_min_max=off  use_precision=off  use_mototune_group=off  data_stores=motohawk_sfun_calibration_data_stores
      settings: SourceProductName=MotoHawk
  motohawk_calibration1 : MotoHawk_lib/Calibration & Probing Blocks/motohawk_calibration  name_source=Use Parameter  nam='U_Bat_Offset'  val=0  storage=Calibration  ovr_cals=on  data_type=Inherit from 'Default Value'  mem_region_use=off  mem_region_name='SERIAL_EE'  read_level=1  write_level=1  view_as=Number  enum_struct={'Disabled', 'Enabled'}  vector_style=Wide Row  row_header_enum={}  col_header_enum={}  mototune_group=motohawk_vardec_path(gcb)  help=''  units=''  min_val=-inf  max_val=inf  precision=''  gain=1  offset=0  exp=1  show_more=off  use_help_units=off  use_header_enum=off  use_min_max=off  use_precision=off  use_mototune_group=off  data_stores=motohawk_sfun_calibration_data_stores
      settings: SourceProductName=MotoHawk
  motohawk_override_abs : MotoHawk_lib/Calibration & Probing Blocks/motohawk_override_abs  parent_name='U_Bat'  parent_val=15  show_more=off  name_source=Use Parameter  parent_read_level=1  parent_override_level=1  view_as=Number  enum_struct={'Disabled', 'Enabled'}  use_help_units=off  parent_help=''  parent_units=''  use_min_max=off  parent_min=-inf  parent_max=inf  use_precision=off  parent_precision=''  parent_gain=1  parent_offset=0  parent_exp=1  use_mototune_group=off  parent_group=motohawk_vardec_path(gcb)
      settings: SourceProductName=MotoHawk
  motohawk_probe : MotoHawk_lib/Calibration & Probing Blocks/motohawk_probe  nam='U_Bat_postc'  show_more=off  name_source=Use Parameter  read_level=1  view_as=Number  enum_struct={'Disabled', 'Enabled'}  vector_style=Wide Row  use_help_units=off  help=''  units=''  use_header_enum=off  row_header_enum={}  col_header_enum={}  use_min_max=off  min_val=-inf  max_val=inf  use_precision=off  precision=''  gain=1  offset=0  exp=1  use_mototune_group=off  mototune_group=motohawk_vardec_path(gcb)
      settings: SourceProductName=MotoHawk
  motohawk_probe1 : MotoHawk_lib/Calibration & Probing Blocks/motohawk_probe  nam='U_Bat'  show_more=off  name_source=Use Parameter  read_level=1  view_as=Number  enum_struct={'Disabled', 'Enabled'}  vector_style=Wide Row  use_help_units=off  help=''  units=''  use_header_enum=off  row_header_enum={}  col_header_enum={}  use_min_max=off  min_val=-inf  max_val=inf  use_precision=off  precision=''  gain=1  offset=0  exp=1  use_mototune_group=off  mototune_group=motohawk_vardec_path(gcb)
      settings: SourceProductName=MotoHawk
  U_Bat : Outport  VectorParamsAs1DForOutWhenUnconnected=off
  wires:
  motohawk_calibration/1 -> Product/2
  Product/1 -> Sum/1
  motohawk_calibration1/1 -> Sum/2
  Gain/1 -> Product/1
  ADC/1 -> Gain/1, motohawk_probe1/1
  Sum/1 -> motohawk_override_abs/1
  motohawk_override_abs/1 -> motohawk_probe/1, U_Bat/1
